simulink model "Sim_13_forh"  (R2019b)
settings: Solver=FixedStepAuto  StartTime=0.0  StopTime=sim_time  FixedStep=0.01  MaxStep=0.1  MinStep=0.0001  RelTol=0.01  AbsTol=0.01
values from neighbouring files (symbols this model uses):
  D = [ 0.66  0    0 ... (first row only)    [Sim_10_init.m]    (also in Sim_11_init.m; Sim_12_init.m; Sim_3_4_and_5_init.m; Sim_7_8_userdef_init.m)
  K_p = 0.08*[1.1  0    0 ... (first row only)    [Sim_10_init.m]    (also in Sim_11_init.m; Sim_12_init.m; Sim_3_4_and_5_init.m; Sim_7_8_userdef_init.m)
  K_v = 1*[10   0       0 ... (first row only)    [Sim_10_init.m]    (also in Sim_11_init.m; Sim_12_init.m; Sim_3_4_and_5_init.m; Sim_7_8_userdef_init.m = 3*[10   0       0)
  L1 = 10*diag([1 1 1])    [Sim_10_init.m]    (also in Sim_11_init.m; Sim_12_init.m; Sim_3_4_and_5_init.m; Sim_7_8_userdef_init.m)
  L2 = 20*M*diag([1 1 1])    [Sim_10_init.m]    (also in Sim_11_init.m; Sim_12_init.m; Sim_3_4_and_5_init.m = 10*M*diag([1 1 1]); Sim_7_8_userdef_init.m)
  L3 = 0.1*L2    [Sim_10_init.m]    (also in Sim_11_init.m; Sim_12_init.m; Sim_3_4_and_5_init.m; Sim_7_8_userdef_init.m)
  M = [ 16    0      0 ... (first row only)    [Sim_10_init.m]    (also in Sim_11_init.m; Sim_12_init.m; Sim_3_4_and_5_init.m; Sim_7_8_userdef_init.m)
  M_1 = inv(M)    [Sim_10_init.m]    (also in Sim_11_init.m; Sim_12_init.m; Sim_3_4_and_5_init.m; Sim_7_8_userdef_init.m)
  mu = 0.09    [Sim_10_init.m]    (also in Sim_11_init.m; Sim_12_init.m; Sim_3_4_and_5_init.m; Sim_7_8_userdef_init.m)
  path_planner_data = [start_pos; end_pos; Radius; Center]    [Sim_10_init.m]    (also in Sim_11_init.m; Sim_12_init.m; Sim_3_4_and_5_init.m; Sim_7_8_userdef_init.m)
  pathparameter = 0    [Sim_10_init.m]    (also in Sim_11_init.m = 1; Sim_12_init.m; Sim_3_4_and_5_init.m = 1; Sim_7_8_userdef_init.m = 1)
  start_pos = [10; 20; pi/2 ]    [Sim_10_init.m]    (also in Sim_11_init.m = [0; 0; 0 ]; Sim_12_init.m = [0; 0; 0 ]; Sim_3_4_and_5_init.m = [0; 0; 0 ]; Sim_7_init.m = [0; 0; 0 ])
undefined symbols (not defined in the file or in its folder): eta_set, p, start_time, t1, t2, t3, time
(part 1 of 3)
settings Model: Creator=einarsu  LastModifiedBy=yngve
settings SolverCC: InitialStep=0.01
settings DataIOCC: ReturnWorkspaceOutputs=off
settings OptimizationCC: LifeSpan=inf
settings DebuggingCC: SFExecutionAtInitializationDiag=none  ArithmeticOperatorsInVariantConditions=warning
settings SFSimCC: SimUseLocalCustomCode=off  CustomCodeUndefinedFunction=UseInterfaceOnly
settings RTWCC: RTWUseLocalCustomCode=off
settings CodeAppCC: StateflowObjectComments=on

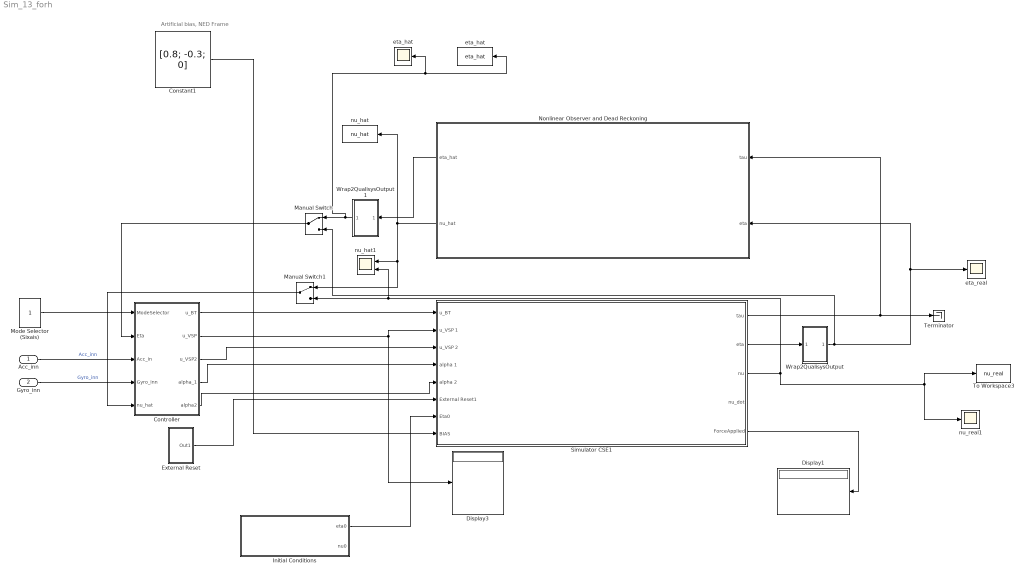
== system Sim_13_forh ==
  note: Artificial bias, NED Frame
  Acc_inn : Inport
  Gyro_inn : Inport  Port=2
  Constant1 : Constant  Value=[0.8; -0.3; 0]
  Controller : Subsystem
  Display1 : Display
  Display3 : Display
  External Reset : Subsystem
  "Initial Conditions " : Subsystem
  Manual Switch : ManualSwitch
  Manual Switch1 : ManualSwitch
  Mode Selector (Sixais) : Constant
  Nonlinear Observer and Dead Reckoning : Subsystem
  Simulator CSE1 : Subsystem
  Terminator : Terminator
  To Workspace3 : ToWorkspace  VariableName=nu_real  SaveFormat=Timeseries  SampleTime=-1
  "Wrap2QualisysOutput " : Subsystem
  Wrap2QualisysOutput 1 : Subsystem
  eta_hat : ToWorkspace  VariableName=eta_hat  SaveFormat=Timeseries  SampleTime=-1
  "eta_hat " : Scope
  "eta_real " : Scope
  nu_hat : ToWorkspace  VariableName=nu_hat  SaveFormat=Structure With Time  SampleTime=-1
  "nu_hat1 " : Scope  NumInputPorts=2
  "nu_real1 " : Scope
  wires:
  Controller/1(u_BT) -> Simulator CSE1/1(u_BT)
  Controller/4(alpha_1) -> Simulator CSE1/4(alpha 1)
  Controller/2(u_VSP) -> Simulator CSE1/2(u_VSP 1), Display3/1
  Controller/5(alpha2) -> Simulator CSE1/5(alpha 2)
  Controller/3("u_VSP2 ") -> Simulator CSE1/3(u_VSP 2)
  External Reset/1(Out1) -> Simulator CSE1/6(External Reset1)
  "Initial Conditions "/1(eta0) -> Simulator CSE1/7(Eta0)
  Mode Selector (Sixais)/1 -> Controller/1(ModeSelector)
  Simulator CSE1/2(eta) -> "Wrap2QualisysOutput "/1(In1)
  Acc_inn/1 -> Controller/3(Acc_in)  "Acc_inn"
  Gyro_inn/1 -> Controller/4(Gyro_inn)  "Gyro_inn"
  Simulator CSE1/5(ForceApplied) -> Display1/1
  Constant1/1 -> Simulator CSE1/8(BIAS)
  Nonlinear Observer and Dead Reckoning/1(eta_hat) -> Wrap2QualisysOutput 1/1(In1)
  Nonlinear Observer and Dead Reckoning/2(nu_hat) -> nu_hat/1, "nu_hat1 "/1, Manual Switch1/1
  Simulator CSE1/3(nu) -> To Workspace3/1, "nu_real1 "/1, Manual Switch1/2, "nu_hat1 "/2
  Simulator CSE1/1(tau) -> Terminator/1, Nonlinear Observer and Dead Reckoning/1(tau)
  "Wrap2QualisysOutput "/1(Out1) -> Manual Switch/2, "eta_real "/1, Nonlinear Observer and Dead Reckoning/2(eta)
  Manual Switch/1 -> Controller/2(Eta)
  Wrap2QualisysOutput 1/1(Out1) -> eta_hat/1, "eta_hat "/1, Manual Switch/1
  Manual Switch1/1 -> Controller/5("nu_hat ")

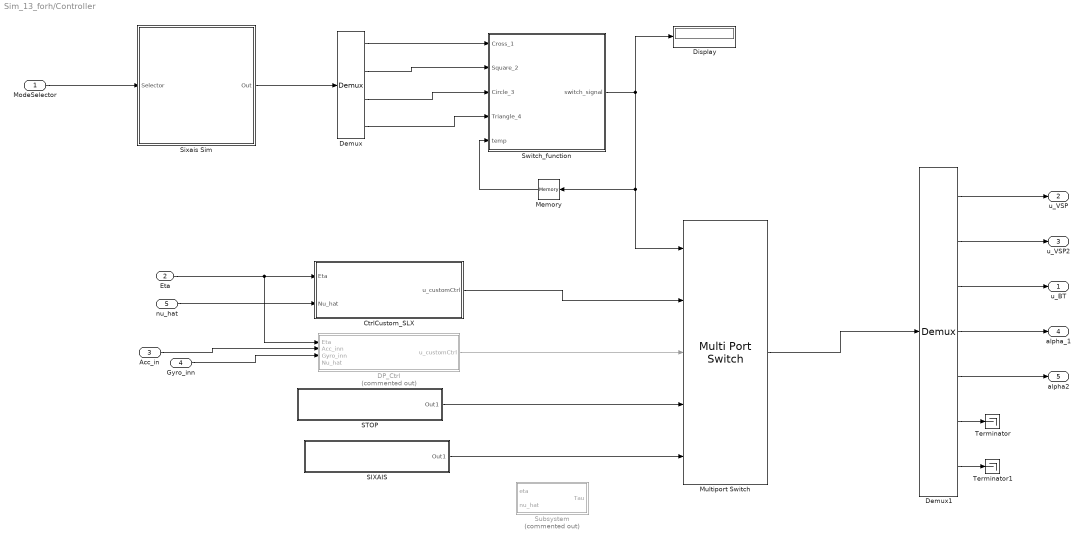
== system Sim_13_forh/Controller ==
  ModeSelector : Inport
  Eta : Inport  Port=2
  Acc_in : Inport  Port=3
  Gyro_inn : Inport  Port=4
  "nu_hat " : Inport  Port=5
  CtrlCustom_SLX : Subsystem
  DP_Ctrl : Subsystem  Commented=on
  Demux : Demux
  Demux1 : Demux  Outputs=7
  Display : Display
  Memory : Memory  InitialCondition=4
  Multiport Switch : MultiPortSwitch  Inputs=4
  SIXAIS : Subsystem
  STOP : Subsystem
  Sixais Sim : MATLAB Function  TreatAsAtomicUnit=on
  Subsystem : Subsystem  Commented=on
  Switch_function : MATLAB Function  TreatAsAtomicUnit=on
  Terminator : Terminator
  Terminator1 : Terminator
  u_BT : Outport  VectorParamsAs1DForOutWhenUnconnected=off
  u_VSP : Outport  Port=2  VectorParamsAs1DForOutWhenUnconnected=off
  "u_VSP2 " : Outport  Port=3  VectorParamsAs1DForOutWhenUnconnected=off
  alpha_1 : Outport  Port=4  VectorParamsAs1DForOutWhenUnconnected=off
  alpha2 : Outport  Port=5  VectorParamsAs1DForOutWhenUnconnected=off
  wires:
  Switch_function/1(switch_signal) -> Multiport Switch/1, Memory/1, Display/1
  Memory/1 -> Switch_function/5(temp)
  CtrlCustom_SLX/1(u_customCtrl) -> Multiport Switch/2
  Demux/1 -> Switch_function/1(Cross_1)
  Demux/2 -> Switch_function/2(Square_2)
  Demux/3 -> Switch_function/3(Circle_3)
  Demux/4 -> Switch_function/4(Triangle_4)
  Sixais Sim/1(Out) -> Demux/1
  ModeSelector/1 -> Sixais Sim/1(Selector)
  DP_Ctrl/1(u_customCtrl) -> Multiport Switch/3
  STOP/1(Out1) -> Multiport Switch/4
  SIXAIS/1(Out1) -> Multiport Switch/5
  Eta/1 -> DP_Ctrl/1(Eta), CtrlCustom_SLX/1(Eta)
  Acc_in/1 -> DP_Ctrl/2(Acc_inn)
  Gyro_inn/1 -> DP_Ctrl/3(Gyro_inn)
  Multiport Switch/1 -> Demux1/1
  Demux1/1 -> u_VSP/1
  Demux1/2 -> "u_VSP2 "/1
  Demux1/3 -> u_BT/1
  Demux1/4 -> alpha_1/1
  Demux1/5 -> alpha2/1
  Demux1/6 -> Terminator/1
  Demux1/7 -> Terminator1/1
  "nu_hat "/1 -> CtrlCustom_SLX/2(Nu_hat)

== system Sim_13_forh/External Reset ==
  note: Most relevant for Real-Time Simulations...
  Constant : Constant  Value=0
  Out1 : Outport  VectorParamsAs1DForOutWhenUnconnected=off
  wires:
  Constant/1 -> Out1/1

== system Sim_13_forh/Initial Conditions  ==
  Eta0 : Constant  Value=start_pos
  "V0 " : Constant  Value=zeros(3,1)
  eta0 : Outport  VectorParamsAs1DForOutWhenUnconnected=off
  nu0 : Outport  Port=2  VectorParamsAs1DForOutWhenUnconnected=off
  wires:
  "V0 "/1 -> nu0/1
  Eta0/1 -> eta0/1

== system Sim_13_forh/Nonlinear Observer and Dead Reckoning ==
  tau : Inport
  eta : Inport  Port=2
  Dead Reckoning : Subsystem
  Nonlinear Observer : Subsystem
  Scope : Scope
  eta_hat : Outport  VectorParamsAs1DForOutWhenUnconnected=off
  nu_hat : Outport  Port=2  VectorParamsAs1DForOutWhenUnconnected=off
  wires:
  Nonlinear Observer/1(eta_hat) -> Dead Reckoning/1(Eta_hat), eta_hat/1  "eta_hat"
  tau/1 -> Nonlinear Observer/2(tau)  "Tau"
  Nonlinear Observer/2(nu_hat) -> nu_hat/1
  Dead Reckoning/1(eta_out) -> Nonlinear Observer/1("eta_out_from_deadreck "), Scope/1
  eta/1 -> Dead Reckoning/2(eta)  "True Eta"

== system Sim_13_forh/Simulator CSE1 ==
  u_BT : Inport
  u_VSP 1 : Inport  Port=2
  u_VSP 2 : Inport  Port=3
  alpha 1 : Inport  Port=4
  alpha 2 : Inport  Port=5
  External Reset1 : Inport  Port=6
  Eta0 : Inport  Port=7
  BIAS : Inport  Port=8
  B Command to force mapping : Subsystem
  Display : Display
  Display1 : Display
  EquationsOfMotion (Fossen Model) : Subsystem
  Mux2 : Mux  Inputs=3
  tau : Outport  VectorParamsAs1DForOutWhenUnconnected=off
  eta : Outport  Port=2  VectorParamsAs1DForOutWhenUnconnected=off
  nu : Outport  Port=3  VectorParamsAs1DForOutWhenUnconnected=off
  nu_dot : Outport  Port=4  VectorParamsAs1DForOutWhenUnconnected=off
  ForceApplied : Outport  Port=5  VectorParamsAs1DForOutWhenUnconnected=off
  wires:
  alpha 2/1 -> B Command to force mapping/5(alpha 2)
  B Command to force mapping/2("F_y ") -> Mux2/2
  B Command to force mapping/1(F_x) -> Mux2/1
  u_VSP 1/1 -> B Command to force mapping/2(u_VSP 1), Display1/1
  alpha 1/1 -> B Command to force mapping/3(alpha 1)
  u_BT/1 -> B Command to force mapping/1(u_BT), Display/1
  u_VSP 2/1 -> B Command to force mapping/6(u_VSP 2)
  EquationsOfMotion (Fossen Model)/2(nuOut) -> B Command to force mapping/4(nu), EquationsOfMotion (Fossen Model)/4(nuInn), nu/1
  Eta0/1 -> EquationsOfMotion (Fossen Model)/1("[eta0] ")
  External Reset1/1 -> EquationsOfMotion (Fossen Model)/2(External Reset)
  EquationsOfMotion (Fossen Model)/1(EtaOut) -> eta/1
  EquationsOfMotion (Fossen Model)/3(nudot) -> nu_dot/1
  B Command to force mapping/3("MOMENT ") -> Mux2/3
  BIAS/1 -> EquationsOfMotion (Fossen Model)/5(Aritifiicial BIas)
  Mux2/1 -> ForceApplied/1, tau/1, EquationsOfMotion (Fossen Model)/3(tau)

== system Sim_13_forh/Wrap2QualisysOutput  ==
  In1 : Inport
  Demux : Demux  Outputs=3
  Gain : Gain  Gain=1000
  Gain1 : Gain  Gain=1000
  Gain2 : Gain  Gain=180/pi
  Mux : Mux  Inputs=3
  Wrap2psi : MATLAB Function  TreatAsAtomicUnit=on
  Out1 : Outport  VectorParamsAs1DForOutWhenUnconnected=off
  wires:
  Mux/1 -> Out1/1
  In1/1 -> Demux/1
  Demux/3 -> Wrap2psi/1(u)
  Demux/1 -> Gain/1
  Demux/2 -> Gain1/1
  Gain/1 -> Mux/1
  Gain1/1 -> Mux/2
  Gain2/1 -> Mux/3
  Wrap2psi/1(yQualisus) -> Gain2/1

== system Sim_13_forh/Wrap2QualisysOutput 1 ==
  In1 : Inport
  Demux : Demux  Outputs=3
  Gain : Gain  Gain=1000
  Gain1 : Gain  Gain=1000
  Gain2 : Gain  Gain=180/pi
  Mux : Mux  Inputs=3
  Wrap2psi : MATLAB Function  TreatAsAtomicUnit=on
  Out1 : Outport  VectorParamsAs1DForOutWhenUnconnected=off
  wires:
  Mux/1 -> Out1/1
  In1/1 -> Demux/1
  Demux/3 -> Wrap2psi/1(u)
  Demux/1 -> Gain/1
  Demux/2 -> Gain1/1
  Gain/1 -> Mux/1
  Gain1/1 -> Mux/2
  Gain2/1 -> Mux/3
  Wrap2psi/1(yQualisus) -> Gain2/1

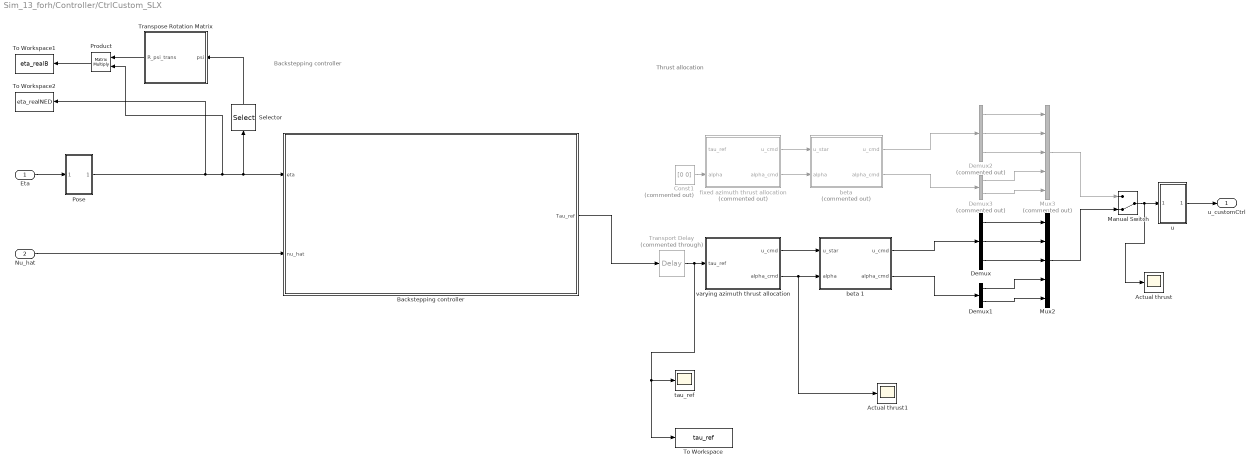
== system Sim_13_forh/Controller/CtrlCustom_SLX ==
  note: Backstepping controller
  note: Thrust allocation
  Eta : Inport
  Nu_hat : Inport  Port=2
  Actual thrust : Scope
  Actual thrust1 : Scope
  Backstepping controller : Subsystem
  Const1 : Constant  Commented=on  Value=[0 0]
  Demux : Demux  Outputs=3
  Demux1 : Demux  Outputs=2
  Demux2 : Demux  Commented=on  Outputs=3
  Demux3 : Demux  Commented=on  Outputs=2
  Manual Switch : ManualSwitch  CurrentSetting=0
  Mux2 : Mux  Inputs=5
  Mux3 : Mux  Commented=on  Inputs=5
  Pose : Subsystem
  Product : Product  Multiplication=Matrix(*)
  Selector : Selector  InputPortWidth=3  IndexOptions=Index vector (dialog)  Indices=[3]  OutputSizes=1
  To Workspace : ToWorkspace  VariableName=tau_ref  SaveFormat=Timeseries  SampleTime=-1
  To Workspace1 : ToWorkspace  VariableName=eta_realB  SaveFormat=Timeseries  SampleTime=-1
  To Workspace2 : ToWorkspace  VariableName=eta_realNED  SaveFormat=Timeseries  SampleTime=-1
  Transport Delay : TransportDelay  Commented=through  DelayTime=50  InitialOutput=[0.1 0.1 0.1]
  Transpose Rotation Matrix : MATLAB Function  TreatAsAtomicUnit=on
  "beta " : MATLAB Function  Commented=on  TreatAsAtomicUnit=on
  beta 1 : MATLAB Function  TreatAsAtomicUnit=on
  "fixed azimuth thrust allocation " : MATLAB Function  Commented=on  TreatAsAtomicUnit=on
  "tau_ref " : Scope
  u : Subsystem
  varying azimuth thrust allocation : MATLAB Function  TreatAsAtomicUnit=on
  u_customCtrl : Outport  VectorParamsAs1DForOutWhenUnconnected=off
  wires:
  u/1(Out1) -> u_customCtrl/1
  Const1/1 -> "fixed azimuth thrust allocation "/2(alpha)
  "fixed azimuth thrust allocation "/2(alpha_cmd) -> "beta "/2(alpha)
  varying azimuth thrust allocation/1(u_cmd) -> beta 1/1(u_star)
  "fixed azimuth thrust allocation "/1(u_cmd) -> "beta "/1(u_star)
  Manual Switch/1 -> Actual thrust/1, u/1(In1)
  beta 1/1(u_cmd) -> Demux/1
  Demux1/2 -> Mux2/5
  beta 1/2(alpha_cmd) -> Demux1/1
  Demux1/1 -> Mux2/4
  Demux/3 -> Mux2/3
  Demux/2 -> Mux2/2
  Demux/1 -> Mux2/1
  Demux3/2 -> Mux3/5
  Demux3/1 -> Mux3/4
  "beta "/2(alpha_cmd) -> Demux3/1
  Demux2/3 -> Mux3/3
  "beta "/1(u_cmd) -> Demux2/1
  Demux2/2 -> Mux3/2
  Demux2/1 -> Mux3/1
  Mux2/1 -> Manual Switch/2
  Mux3/1 -> Manual Switch/1
  Nu_hat/1 -> Backstepping controller/2(nu_hat)
  Pose/1(QTM) -> To Workspace2/1, Product/2, Selector/1, Backstepping controller/1(eta)
  Transpose Rotation Matrix/1(R_psi_trans) -> Product/1
  Product/1 -> To Workspace1/1
  Eta/1 -> Pose/1(eta)
  Selector/1 -> Transpose Rotation Matrix/1(psi)
  varying azimuth thrust allocation/2(alpha_cmd) -> Actual thrust1/1, beta 1/2(alpha)
  Backstepping controller/1("Tau_ref ") -> Transport Delay/1
  Transport Delay/1 -> To Workspace/1, "tau_ref "/1, varying azimuth thrust allocation/1(tau_ref)

== system Sim_13_forh/Controller/DP_Ctrl ==
  Eta : Inport
  Acc_inn : Inport  Port=2
  Gyro_inn : Inport  Port=3
  Nu_hat : Inport  Port=4
  Backstepping controller : Subsystem
  Constant : Constant  Value=[1;0;0]
  IMU (Consider if going to be properly Simulated...) : Subsystem
  Manual Switch : ManualSwitch  CurrentSetting=0
  Pose : Subsystem
  "Thrust Allocation " : Subsystem
  u : Subsystem
  u_customCtrl : Outport  VectorParamsAs1DForOutWhenUnconnected=off
  wires:
  Gyro_inn/1 -> IMU (Consider if going to be properly Simulated...)/1(Gyro_inn)
  Acc_inn/1 -> IMU (Consider if going to be properly Simulated...)/2(Acc_inn)
  Eta/1 -> Pose/1(eta)
  u/1(Out1) -> u_customCtrl/1
  IMU (Consider if going to be properly Simulated...)/2(Gyro) -> ?
  IMU (Consider if going to be properly Simulated...)/1(Acc) -> ?
  Constant/1 -> Manual Switch/1
  Manual Switch/1 -> "Thrust Allocation "/1(Tau_ref)
  "Thrust Allocation "/1(u_customCtrl) -> u/1(In1)
  Nu_hat/1 -> Backstepping controller/2(nu_hat)
  Pose/1(QTM) -> Backstepping controller/1(eta)
  Backstepping controller/1(Tau) -> Manual Switch/2

== system Sim_13_forh/Controller/SIXAIS ==
  Constant{,1..6} (7 alike) : Constant  Value=0
  Sixais Controller Not Simulated in Simulink : Subsystem
  Out1 : Outport  VectorParamsAs1DForOutWhenUnconnected=off
  wires:
  Constant/1 -> Sixais Controller Not Simulated in Simulink/1(In1)
  Constant1/1 -> Sixais Controller Not Simulated in Simulink/2(In2)
  Constant2/1 -> Sixais Controller Not Simulated in Simulink/3(In3)
  Constant3/1 -> Sixais Controller Not Simulated in Simulink/4(In4)
  Constant4/1 -> Sixais Controller Not Simulated in Simulink/5(In5)
  Constant5/1 -> Sixais Controller Not Simulated in Simulink/6(In6)
  Constant6/1 -> Sixais Controller Not Simulated in Simulink/7(In7)
  Sixais Controller Not Simulated in Simulink/1(Out1) -> Out1/1

== system Sim_13_forh/Controller/STOP ==
  Constant{,1..6} (7 alike) : Constant  Value=0
  Mux1 : Mux  Inputs=7
  Out1 : Outport  VectorParamsAs1DForOutWhenUnconnected=off
  wires:
  Mux1/1 -> Out1/1
  Constant/1 -> Mux1/1
  Constant1/1 -> Mux1/2
  Constant2/1 -> Mux1/3
  Constant3/1 -> Mux1/4
  Constant4/1 -> Mux1/5
  Constant5/1 -> Mux1/6
  Constant6/1 -> Mux1/7

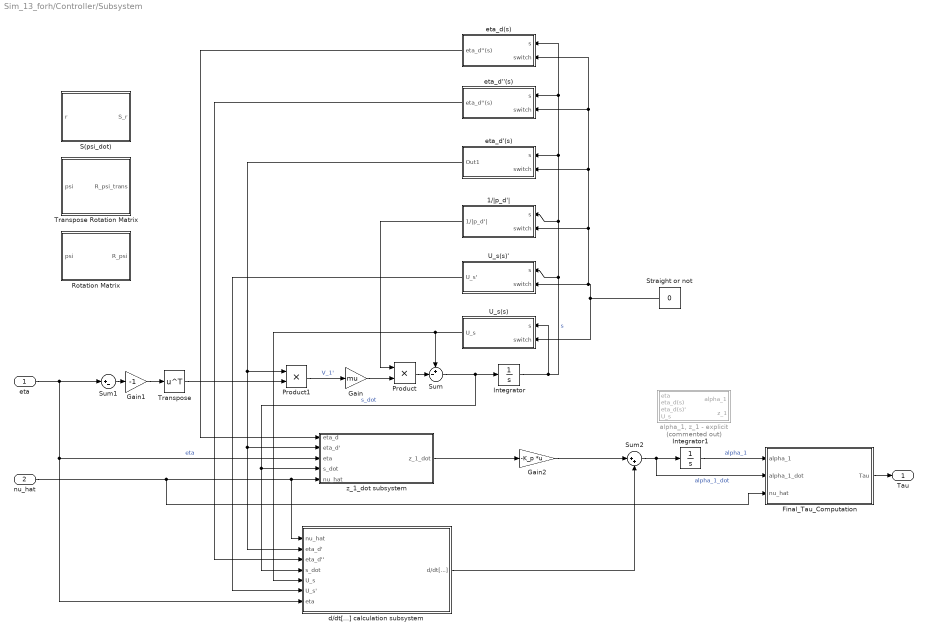
== system Sim_13_forh/Controller/Subsystem ==
  eta : Inport
  nu_hat : Inport  Port=2
  1/|p_d'| : Subsystem
  Final_Tau_Computation : Subsystem
  Gain : Gain  Gain=mu
  Gain1 : Gain  Gain=-1
  Gain2 : Gain  Gain=-K_p  Multiplication=Matrix(K*u)
  Integrator : Integrator
  Integrator1 : Integrator
  Product : Product
  Product1 : Product
  Rotation Matrix : MATLAB Function  TreatAsAtomicUnit=on
  S(psi_dot) : MATLAB Function  TreatAsAtomicUnit=on
  Straight or not : Constant  Value=0
  Sum : Sum  Inputs=+-|
  Sum1 : Sum  Inputs=|+-
  Sum2 : Sum  Inputs=|++
  Transpose : Math  Operator=transpose  SignedPower=off  SaturateOnIntegerOverflow=on
  Transpose Rotation Matrix : MATLAB Function  TreatAsAtomicUnit=on
  U_s(s) : Subsystem
  U_s(s)' : Subsystem
  "alpha_1, z_1 - explicit " : Subsystem  Commented=on
  d/dt[...] calculation subsystem : Subsystem
  eta_d''(s) : Subsystem
  eta_d'(s) : Subsystem
  eta_d(s) : Subsystem
  "z_1_dot subsystem " : Subsystem
  Tau : Outport
  wires:
  Integrator/1 -> U_s(s)'/1(s), 1/|p_d'|/1(s), eta_d'(s)/1(s), eta_d(s)/1(s), eta_d''(s)/1(s), U_s(s)/1(s)  "s"
  Sum/1 -> "z_1_dot subsystem "/4(s_dot), d/dt[...] calculation subsystem/4(s_dot), Integrator/1  "s_dot"
  U_s(s)/1(U_s) -> Sum/1, d/dt[...] calculation subsystem/5(U_s)
  Gain/1 -> Product/2
  Product/1 -> Sum/2
  1/|p_d'|/1(1/|p_d'|) -> Product/1
  eta_d'(s)/1(Out1) -> Product1/1, d/dt[...] calculation subsystem/2(eta_d'), "z_1_dot subsystem "/2(eta_d')
  Product1/1 -> Gain/1  "V_1'"
  Sum1/1 -> Gain1/1
  eta/1 -> "z_1_dot subsystem "/3(eta), d/dt[...] calculation subsystem/7("eta "), Sum1/1  "eta"
  ? -> Sum1/2  "eta_d"
  Gain1/1 -> Transpose/1
  Transpose/1 -> Product1/2
  "z_1_dot subsystem "/1(z_1_dot) -> Gain2/1
  Gain2/1 -> Sum2/1
  d/dt[...] calculation subsystem/1(d/dt[...]) -> Sum2/2
  Sum2/1 -> Final_Tau_Computation/2(alpha_1_dot), Integrator1/1  "alpha_1_dot"
  nu_hat/1 -> Final_Tau_Computation/3(nu_hat), d/dt[...] calculation subsystem/1(nu_hat), "z_1_dot subsystem "/5(nu_hat)
  Integrator1/1 -> Final_Tau_Computation/1(alpha_1)  "alpha_1"
  Final_Tau_Computation/1(Tau) -> Tau/1
  U_s(s)'/1(U_s') -> d/dt[...] calculation subsystem/6("U_s' ")
  Straight or not/1 -> U_s(s)/2(switch), eta_d(s)/2(switch), eta_d''(s)/2(switch), eta_d'(s)/2(switch), 1/|p_d'|/2(switch), U_s(s)'/2("switch ")
  eta_d''(s)/1("eta_d''(s) ") -> d/dt[...] calculation subsystem/3(eta_d'')
  eta_d(s)/1("eta_d''(s) ") -> "z_1_dot subsystem "/1(eta_d)

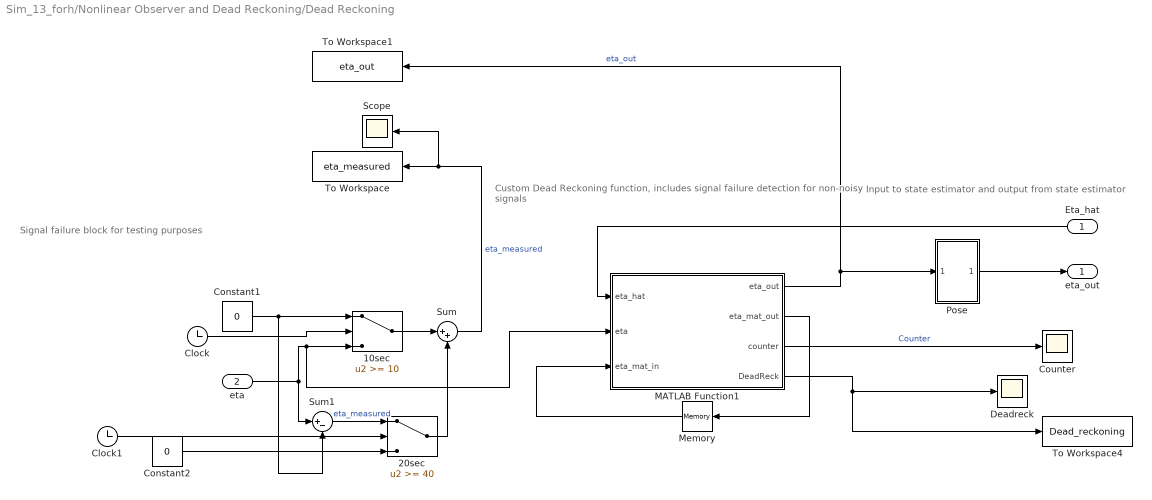
== system Sim_13_forh/Nonlinear Observer and Dead Reckoning/Dead Reckoning ==
  note: Custom Dead Reckoning function, includes signal failure
      | detection for non-noisy signals
  note: Input to state estimator and output from state estimator
  note: Signal failure block for testing purposes
  Eta_hat : Inport
  eta : Inport  Port=2
  10sec : Switch  Threshold=10
  "20sec " : Switch  Threshold=40
  Clock : Clock
  Clock1 : Clock
      settings: Decimation=20
  Constant1 : Constant  Value=0
  Constant2 : Constant  Value=0
  Counter : Scope
  "Deadreck " : Scope
  MATLAB Function1 : MATLAB Function  TreatAsAtomicUnit=on
  Memory : Memory  InitialCondition=zeros(4,3)  InheritSampleTime=on
  Pose : Subsystem
  Scope : Scope
  Sum : Sum  Inputs=|++
  Sum1 : Sum  Inputs=|+-
  To Workspace : ToWorkspace  VariableName=eta_measured  SaveFormat=Timeseries  SampleTime=-1
  To Workspace1 : ToWorkspace  VariableName=eta_out  SampleTime=-1
  To Workspace4 : ToWorkspace  VariableName=Dead_reckoning  SaveFormat=Timeseries  SampleTime=-1
  eta_out : Outport
  wires:
  MATLAB Function1/2(eta_mat_out) -> Memory/1
  Sum/1 -> Scope/1, To Workspace/1  "eta_measured"
  Eta_hat/1 -> MATLAB Function1/1(eta_hat)
  MATLAB Function1/1(eta_out) -> Pose/1(eta), To Workspace1/1  "eta_out"
  Clock1/1 -> "20sec "/2
  Constant1/1 -> Sum1/2, 10sec/1
  Constant2/1 -> "20sec "/3
  MATLAB Function1/4(DeadReck) -> To Workspace4/1, "Deadreck "/1
  "20sec "/1 -> Sum/2
  10sec/1 -> Sum/1
  Memory/1 -> MATLAB Function1/3(eta_mat_in)
  Clock/1 -> 10sec/2
  MATLAB Function1/3(counter) -> Counter/1  "Counter"
  eta/1 -> Sum1/1, MATLAB Function1/2(eta), 10sec/3
  Sum1/1 -> "20sec "/1  "eta_measured"
  Pose/1(QTM) -> eta_out/1

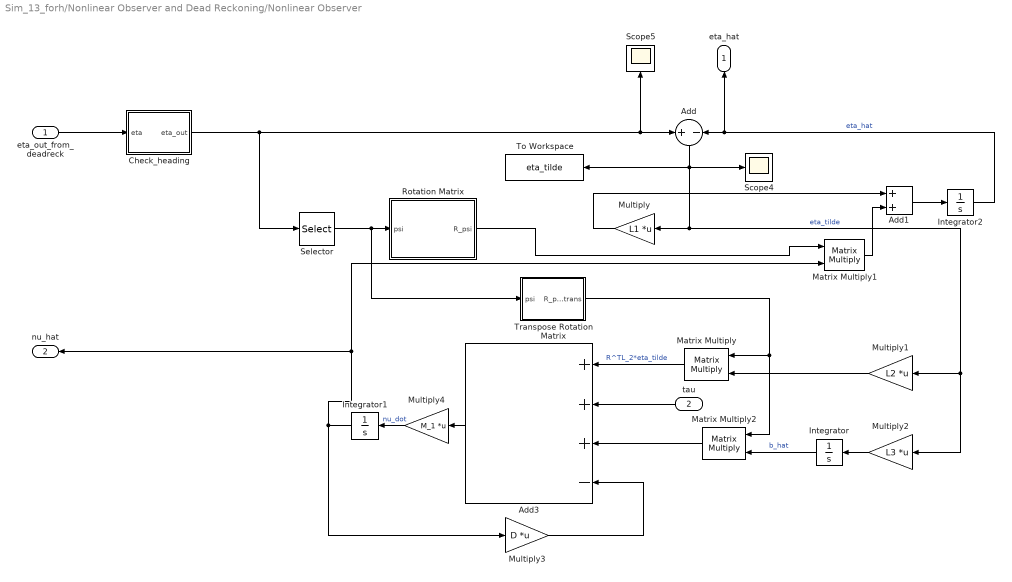
== system Sim_13_forh/Nonlinear Observer and Dead Reckoning/Nonlinear Observer ==
  "eta_out_from_deadreck " : Inport
  tau : Inport  Port=2
  Add : Sum  Inputs=+-
  Add1 : Sum
  Add3 : Sum  Inputs=+++-
  Check_heading : MATLAB Function  TreatAsAtomicUnit=on
  Integrator : Integrator
  Integrator1 : Integrator
  Integrator2 : Integrator
  Matrix Multiply : Product  Multiplication=Matrix(*)
  Matrix Multiply1 : Product  Multiplication=Matrix(*)
  Matrix Multiply2 : Product  Multiplication=Matrix(*)
  Multiply : Gain  Gain=L1  Multiplication=Matrix(K*u)
  Multiply1 : Gain  Gain=L2  Multiplication=Matrix(K*u)
  Multiply2 : Gain  Gain=L3  Multiplication=Matrix(K*u)
  Multiply3 : Gain  Gain=D  Multiplication=Matrix(K*u)
  Multiply4 : Gain  Gain=M_1  Multiplication=Matrix(K*u)
  Rotation Matrix : MATLAB Function  TreatAsAtomicUnit=on
  Scope4 : Scope
  Scope5 : Scope
  Selector : Selector  InputPortWidth=3  IndexOptions=Index vector (dialog)  Indices=3  OutputSizes=1
  To Workspace : ToWorkspace  VariableName=eta_tilde  SaveFormat=Timeseries  SampleTime=-1
  Transpose Rotation Matrix : MATLAB Function  TreatAsAtomicUnit=on
  eta_hat : Outport
  nu_hat : Outport  Port=2  VectorParamsAs1DForOutWhenUnconnected=off
  wires:
  Multiply/1 -> Add1/1
  Multiply2/1 -> Integrator/1
  Rotation Matrix/1(R_psi) -> Matrix Multiply1/1
  Multiply1/1 -> Matrix Multiply/2
  Matrix Multiply/1 -> Add3/1  "R^TL_2*eta_tilde"
  "eta_out_from_deadreck "/1 -> Check_heading/1(eta)
  Matrix Multiply1/1 -> Add1/2
  Add/1 -> Scope4/1, Multiply/1, Multiply1/1, Multiply2/1, To Workspace/1  "eta_tilde"
  Multiply4/1 -> Integrator1/1  "nu_dot"
  Selector/1 -> Transpose Rotation Matrix/1(psi), Rotation Matrix/1(psi)
  Integrator2/1 -> Add/2, eta_hat/1  "eta_hat"
  Integrator/1 -> Matrix Multiply2/2  "b_hat"
  tau/1 -> Add3/2
  Matrix Multiply2/1 -> Add3/3
  Multiply3/1 -> Add3/4
  Add3/1 -> Multiply4/1
  Add1/1 -> Integrator2/1
  Integrator1/1 -> nu_hat/1, Matrix Multiply1/2, Multiply3/1
  Transpose Rotation Matrix/1(R_psi_trans) -> Matrix Multiply2/1, Matrix Multiply/1
  Check_heading/1(eta_out) -> Selector/1, Scope5/1, Add/1

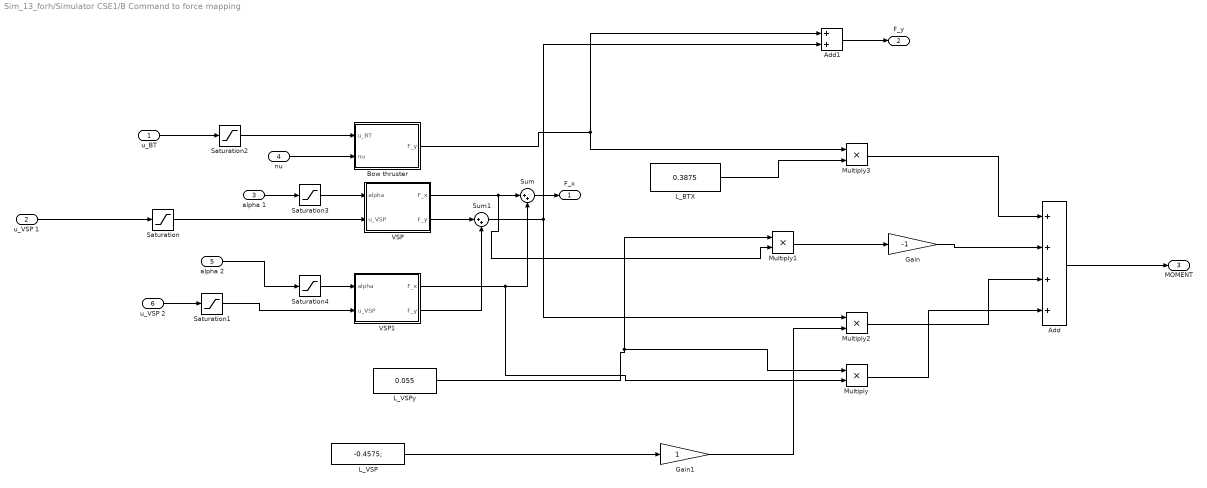
== system Sim_13_forh/Simulator CSE1/B Command to force mapping ==
  u_BT : Inport
  u_VSP 1 : Inport  Port=2
  alpha 1 : Inport  Port=3
  nu : Inport  Port=4
  alpha 2 : Inport  Port=5
  u_VSP 2 : Inport  Port=6
  Add : Sum  Inputs=++++
  Add1 : Sum
  Bow thruster : MATLAB Function  TreatAsAtomicUnit=on
  Gain : Gain  Gain=-1
  Gain1 : Gain
  L_BTX : Constant  Value=0.3875
  L_VSP : Constant  Value=-0.4575;
  L_VSPy : Constant  Value=0.055
  Multiply{,1..3} (4 alike) : Product
  Saturation : Saturate  UpperLimit=1  LowerLimit=0
  Saturation1 : Saturate  UpperLimit=1  LowerLimit=0
  Saturation2 : Saturate  UpperLimit=1  LowerLimit=-1
  Saturation3 : Saturate  UpperLimit=pi  LowerLimit=-pi
  Saturation4 : Saturate  UpperLimit=pi  LowerLimit=-pi
  Sum : Sum  Inputs=|++
  Sum1 : Sum  Inputs=|++
  VSP : MATLAB Function  TreatAsAtomicUnit=on
  VSP1 : MATLAB Function  TreatAsAtomicUnit=on
  F_x : Outport  VectorParamsAs1DForOutWhenUnconnected=off
  "F_y " : Outport  Port=2  VectorParamsAs1DForOutWhenUnconnected=off
  "MOMENT " : Outport  Port=3  VectorParamsAs1DForOutWhenUnconnected=off
  wires:
  alpha 1/1 -> Saturation3/1
  nu/1 -> Bow thruster/2(nu)
  Bow thruster/1(F_y) -> Add1/1, Multiply3/1
  VSP/2(F_y) -> Sum1/1
  Sum1/1 -> Add1/2, Multiply2/1
  VSP1/2(F_y) -> Sum1/2
  VSP1/1(F_x) -> Multiply/2, Sum/2
  VSP/1(F_x) -> Multiply1/2, Sum/1
  Sum/1 -> F_x/1
  alpha 2/1 -> Saturation4/1
  u_VSP 2/1 -> Saturation1/1
  L_VSP/1 -> Gain1/1
  L_BTX/1 -> Multiply3/2
  L_VSPy/1 -> Multiply/1, Multiply1/1
  Multiply3/1 -> Add/1
  Multiply1/1 -> Gain/1
  Multiply2/1 -> Add/3
  Multiply/1 -> Add/4
  Add/1 -> "MOMENT "/1
  Gain/1 -> Add/2
  Gain1/1 -> Multiply2/2
  Add1/1 -> "F_y "/1
  Saturation/1 -> VSP/2(u_VSP)
  Saturation1/1 -> VSP1/2(u_VSP)
  u_BT/1 -> Saturation2/1
  u_VSP 1/1 -> Saturation/1
  Saturation2/1 -> Bow thruster/1(u_BT)
  Saturation3/1 -> VSP/1(alpha)
  Saturation4/1 -> VSP1/1(alpha)

== system Sim_13_forh/Simulator CSE1/EquationsOfMotion (Fossen Model) ==
  "[eta0] " : Inport
  External Reset : Inport  Port=2
  tau : Inport  Port=3
  nuInn : Inport  Port=4
  Aritifiicial BIas : Inport  Port=5
  Add : Sum
  MATLAB Function : MATLAB Function  TreatAsAtomicUnit=on
  Position : Integrator  ExternalReset=either  InitialConditionSource=external  InitialCondition=[0 0 0]'
  Selector : Selector  InputPortWidth=3  IndexOptions=Index vector (dialog)  Indices=[3]  OutputSizes=1
  Velocity : Integrator  ExternalReset=either  InitialCondition=[0 0 0]'
  kinematics : MATLAB Function  TreatAsAtomicUnit=on
  kinetics : MATLAB Function  TreatAsAtomicUnit=on
  EtaOut : Outport  VectorParamsAs1DForOutWhenUnconnected=off
  nuOut : Outport  Port=2  VectorParamsAs1DForOutWhenUnconnected=off
  nudot : Outport  Port=3  VectorParamsAs1DForOutWhenUnconnected=off
  wires:
  tau/1 -> Add/1
  Position/1 -> EtaOut/1, Selector/1, kinematics/2(eta)
  "[eta0] "/1 -> Position/3
  nuInn/1 -> kinetics/2(nu)
  kinematics/1(eta_dot) -> Position/1
  Velocity/1 -> nuOut/1, kinematics/1(nu)
  kinetics/1(nu_dot) -> nudot/1, Velocity/1
  External Reset/1 -> Velocity/2, Position/2
  Add/1 -> kinetics/1(tau)
  Aritifiicial BIas/1 -> MATLAB Function/2(NedVector)
  Selector/1 -> MATLAB Function/1(psi)
  MATLAB Function/1(BodyVector) -> Add/2

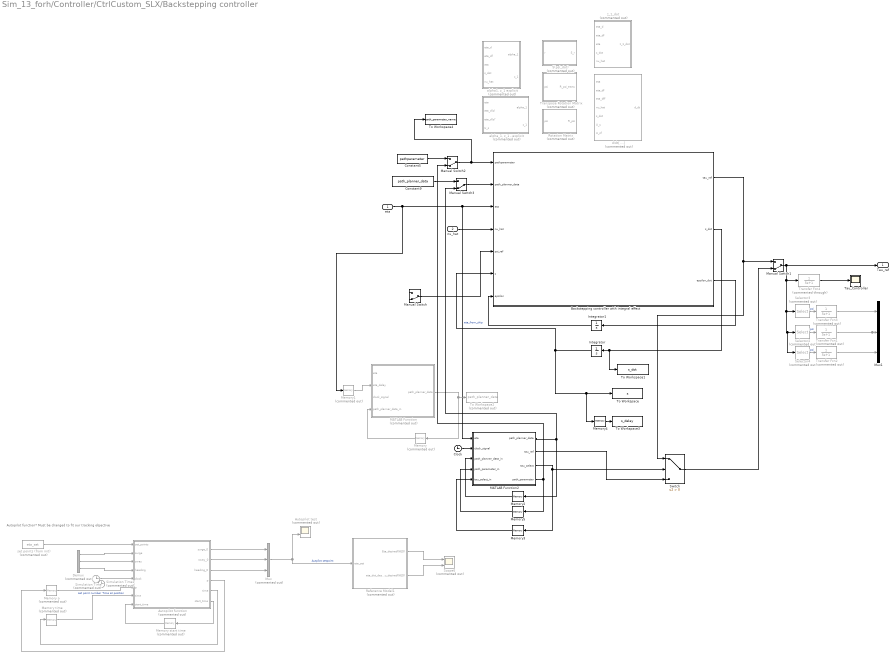
== system Sim_13_forh/Controller/CtrlCustom_SLX/Backstepping controller ==
  note: Autopilot function* Must be changed to fit our tracking objective
  eta : Inport
  nu_hat : Inport  Port=2
  "Autopilot function " : MATLAB Function  Commented=on  TreatAsAtomicUnit=on
  "Autopilot test " : Scope  Commented=on  NumInputPorts=2
  "Backstepping controller with integral effect " : MATLAB Function  TreatAsAtomicUnit=on  SystemSampleTime=0.1
  Clock : Clock
  Constant5 : Constant  Value=pathparameter
  Constant9 : Constant  Value=path_planner_data
  Demux : Demux  Commented=on  Outputs=3
  Integrator : Integrator
  Integrator1 : Integrator  InitialCondition=[0;0;0]  LimitOutput=on  UpperSaturationLimit=1  LowerSaturationLimit=-1
  MATLAB Function : MATLAB Function  Commented=on  TreatAsAtomicUnit=on
  MATLAB Function2 : MATLAB Function  TreatAsAtomicUnit=on
  Manual Switch{,1..3} (4 alike) : ManualSwitch  CurrentSetting=0
  Memory : Memory  Commented=on
  Memory start time : Memory  Commented=on  InitialCondition=start_time  InheritSampleTime=on
  Memory p : Memory  Commented=on  InitialCondition=p  InheritSampleTime=on
  Memory time : Memory  Commented=on  InitialCondition=time
  Memory1 : Memory  Commented=on
  Memory{2..5} (4 alike) : Memory
  Mux : Mux  Commented=on  Inputs=3
  Mux1 : Mux  Inputs=3
  Reference Model1 : Subsystem  Commented=on
  Rotation Matrix : MATLAB Function  Commented=on  TreatAsAtomicUnit=on
  S(psi_dot) : MATLAB Function  Commented=on  TreatAsAtomicUnit=on
  Scope6 : Scope  Commented=on  NumInputPorts=2
  Selector2 : Selector  Commented=on  InputPortWidth=3  IndexOptions=Index vector (dialog)  Indices=[2]  OutputSizes=1
  Selector3 : Selector  Commented=on  InputPortWidth=3  IndexOptions=Index vector (dialog)  Indices=[1]  OutputSizes=1
  Selector4 : Selector  Commented=on  InputPortWidth=3  IndexOptions=Index vector (dialog)  Indices=[3]  OutputSizes=1
  Simulation Time : Clock  Commented=on
  Simulation Time1 : Clock  Commented=on
  Switch : Switch  Criteria=u2 > Threshold
  Tau_Controller : Scope
  To Workspace : ToWorkspace  VariableName=s  SaveFormat=Timeseries  SampleTime=-1
  To Workspace1 : ToWorkspace  VariableName=s_dot  SaveFormat=Timeseries  SampleTime=-1
  To Workspace2 : ToWorkspace  Commented=on  VariableName=path_planner_data  SaveFormat=Timeseries  SampleTime=-1
  To Workspace3 : ToWorkspace  VariableName=s_delay  SaveFormat=Timeseries  SampleTime=-1
  To Workspace4 : ToWorkspace  VariableName=path_parameter_name  SaveFormat=Timeseries  SampleTime=-1
  Transfer Fcn1 : TransferFcn  Commented=on  Denominator=[5 1]
  Transfer Fcn2 : TransferFcn  Commented=on  Denominator=[5 1]
  Transfer Fcn3 : TransferFcn  Commented=on  Denominator=[5 1]
  Transfer Fcn4 : TransferFcn  Commented=through  Denominator=[5 1]
  Transpose Rotation Matrix : MATLAB Function  Commented=on  TreatAsAtomicUnit=on
  "alpha1, z_1 explicit" : MATLAB Function  Commented=on  TreatAsAtomicUnit=on
  "alpha_1, z_1 - explicit " : Subsystem  Commented=on
  d/dt[....] : MATLAB Function  Commented=on  TreatAsAtomicUnit=on
  set points (from init) : Constant  Commented=on  Value=eta_set
  z_1_dot : MATLAB Function  Commented=on  TreatAsAtomicUnit=on
  "Tau_ref " : Outport
  wires:
  Constant9/1 -> Manual Switch3/1
  "Autopilot function "/6(start_time) -> Memory start time/1
  Memory time/1 -> "Autopilot function "/7("time ")  "Time at position"
  Memory start time/1 -> "Autopilot function "/8("start_time ")
  "Autopilot function "/3(heading_0) -> Mux/3
  "Autopilot function "/5(time) -> Memory time/1
  "Autopilot function "/1(surge_0) -> Mux/1
  Simulation Time/1 -> "Autopilot function "/5(clock)
  Demux/2 -> "Autopilot function "/3(sway)
  Demux/1 -> "Autopilot function "/2(surge)
  eta/1 -> Memory1/1, MATLAB Function2/1(eta), "Backstepping controller with integral effect "/3(eta)  "eta_from_ship"
  Demux/3 -> "Autopilot function "/4(heading)
  set points (from init)/1 -> "Autopilot function "/1(set_points)
  "Autopilot function "/2(sway_0) -> Mux/2
  "Autopilot function "/4(p) -> Memory p/1
  Mux/1 -> "Autopilot test "/2, Reference Model1/1("eta_set ")  "Autpilot setpoint"
  Memory p/1 -> "Autopilot function "/6("p ")  "set point number"
  Reference Model1/1(Eta_desired(NED)) -> Scope6/1
  Reference Model1/2(eta_dot_desired = nu_desired(NED)) -> Scope6/2
  Manual Switch1/1 -> Selector3/1, Selector2/1, Selector4/1, Transfer Fcn4/1, "Tau_ref "/1
  Manual Switch3/1 -> "Backstepping controller with integral effect "/2(path_planner_data)
  "Backstepping controller with integral effect "/3(epsilon_dot) -> Integrator1/1
  "Backstepping controller with integral effect "/2(s_dot) -> To Workspace1/1, Integrator/1
  Manual Switch/1 -> "Backstepping controller with integral effect "/5(psi_ref)
  nu_hat/1 -> "Backstepping controller with integral effect "/4(nu_hat)
  Integrator/1 -> Memory4/1, To Workspace/1, "Backstepping controller with integral effect "/6(s)
  Integrator1/1 -> "Backstepping controller with integral effect "/7(epsilon)
  Transfer Fcn1/1 -> Mux1/2
  Selector2/1 -> Transfer Fcn1/1  "psi"
  Selector4/1 -> Transfer Fcn2/1  "psi"
  Selector3/1 -> Transfer Fcn3/1  "psi"
  Transfer Fcn3/1 -> Mux1/1
  Transfer Fcn2/1 -> Mux1/3
  Transfer Fcn4/1 -> Tau_Controller/1
  MATLAB Function/1(path_planner_data) -> To Workspace2/1, Memory/1
  Memory/1 -> MATLAB Function/4(path_planner_data_in)
  Memory1/1 -> MATLAB Function/2(eta_delay)
  Clock/1 -> MATLAB Function2/2(clock_signal)
  MATLAB Function2/1(path_planner_data) -> Manual Switch3/2, Memory2/1
  Memory2/1 -> MATLAB Function2/3(path_planner_data_in)
  MATLAB Function2/3(tau_select) -> Memory3/1, Switch/2
  Memory3/1 -> MATLAB Function2/5(tau_select_in)
  MATLAB Function2/2(tau_ref) -> Switch/3
  "Backstepping controller with integral effect "/1(tau_ref) -> Manual Switch1/1, Switch/1
  Switch/1 -> Manual Switch1/2
  Memory4/1 -> To Workspace3/1
  MATLAB Function2/4(path_parameter) -> Memory5/1, Manual Switch2/2
  Constant5/1 -> Manual Switch2/1
  Manual Switch2/1 -> To Workspace4/1, "Backstepping controller with integral effect "/1(pathparameter)
  Memory5/1 -> MATLAB Function2/4(path_parameter_in)

== system Sim_13_forh/Controller/CtrlCustom_SLX/Pose ==
  eta : Inport
  Demux : Demux  Outputs=3
  Gain : Gain  Gain=1/1000
  Gain1 : Gain  Gain=1/1000
  Gain2 : Gain  Gain=180/pi
  Gain3 : Gain  Gain=pi/180
  MATLAB Function : MATLAB Function  Commented=on  TreatAsAtomicUnit=on
  Manual Switch : ManualSwitch
  Memory : Memory  Commented=on
  Mux : Mux  Inputs=3
  Wrap2psi : MATLAB Function  TreatAsAtomicUnit=on
  QTM : Outport  VectorParamsAs1DForOutWhenUnconnected=off
  wires:
  Demux/2 -> Gain1/1  "y_m"
  Demux/3 -> Gain3/1  "psi_m"
  Demux/1 -> Gain/1  "x_m"
  Mux/1 -> QTM/1
  eta/1 -> Demux/1
  ? -> Wrap2psi/1(u)
  Wrap2psi/1(yQualisus) -> Gain2/1
  Gain/1 -> Mux/1
  Gain1/1 -> Mux/2
  MATLAB Function/1(psi_out) -> Memory/1, Manual Switch/2
  Memory/1 -> MATLAB Function/2(psi_old)
  Gain3/1 -> MATLAB Function/1(psi), Manual Switch/1
  Manual Switch/1 -> Mux/3

== system Sim_13_forh/Controller/CtrlCustom_SLX/u ==
  In1 : Inport
  Constant : Constant  Value=0.3
  Constant1 : Constant  Value=0.3
  Demux1 : Demux  Outputs=5
  Mux : Mux  Inputs=7
  Saturation1 : Saturate  UpperLimit=1  LowerLimit=0
  Saturation11 : Saturate  UpperLimit=1  LowerLimit=0
  Out1 : Outport  VectorParamsAs1DForOutWhenUnconnected=off
  wires:
  In1/1 -> Demux1/1
  Demux1/1 -> Saturation11/1  "u_vsp1"
  Demux1/2 -> Saturation1/1  "u_VSP2"
  Demux1/3 -> Mux/3  "U_BT"
  Demux1/4 -> Mux/4  "alpha_VSP1"
  Demux1/5 -> Mux/5  "alpha_VSP2"
  Constant/1 -> Mux/6  "omega_VSP1"
  Constant1/1 -> Mux/7  "omega_VSP2"
  Mux/1 -> Out1/1
  Saturation11/1 -> Mux/1
  Saturation1/1 -> Mux/2

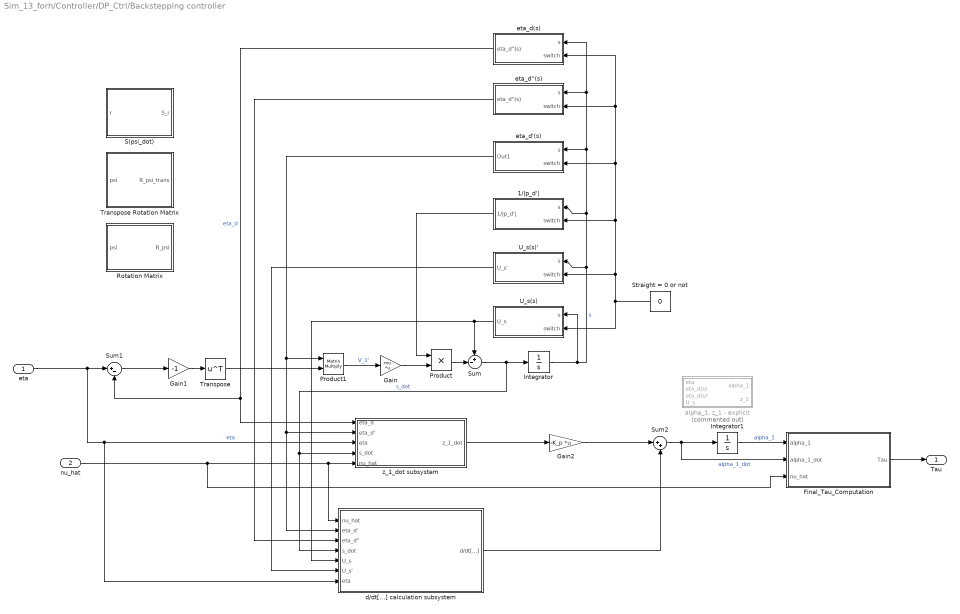
== system Sim_13_forh/Controller/DP_Ctrl/Backstepping controller ==
  eta : Inport
  nu_hat : Inport  Port=2
  1/|p_d'| : Subsystem
  Final_Tau_Computation : Subsystem
  Gain : Gain  Gain=mu  Multiplication=Matrix(K*u)
  Gain1 : Gain  Gain=-1
  Gain2 : Gain  Gain=-K_p  Multiplication=Matrix(K*u)
  Integrator : Integrator
  Integrator1 : Integrator
  Product : Product
  Product1 : Product  Multiplication=Matrix(*)
  Rotation Matrix : MATLAB Function  TreatAsAtomicUnit=on
  S(psi_dot) : MATLAB Function  TreatAsAtomicUnit=on
  Straight = 0 or not : Constant  Value=0
  Sum : Sum  Inputs=+-|
  Sum1 : Sum  Inputs=|+-
  Sum2 : Sum  Inputs=|++
  Transpose : Math  Operator=transpose  SignedPower=off  SaturateOnIntegerOverflow=on
  Transpose Rotation Matrix : MATLAB Function  TreatAsAtomicUnit=on
  U_s(s) : Subsystem
  U_s(s)' : Subsystem
  "alpha_1, z_1 - explicit " : Subsystem  Commented=on
  d/dt[...] calculation subsystem : Subsystem
  eta_d''(s) : Subsystem
  eta_d'(s) : Subsystem
  eta_d(s) : Subsystem
  "z_1_dot subsystem " : Subsystem
  Tau : Outport
  wires:
  Integrator/1 -> U_s(s)'/1(s), 1/|p_d'|/1(s), eta_d'(s)/1(s), eta_d(s)/1(s), eta_d''(s)/1(s), U_s(s)/1(s)  "s"
  Sum/1 -> "z_1_dot subsystem "/4(s_dot), d/dt[...] calculation subsystem/4(s_dot), Integrator/1  "s_dot"
  U_s(s)/1(U_s) -> d/dt[...] calculation subsystem/5(U_s), Sum/1
  Gain/1 -> Product/2
  Product/1 -> Sum/2
  1/|p_d'|/1(1/|p_d'|) -> Product/1
  Product1/1 -> Gain/1  "V_1'"
  Sum1/1 -> Gain1/1
  eta/1 -> Sum1/1, "z_1_dot subsystem "/3(eta), d/dt[...] calculation subsystem/7("eta ")  "eta"
  eta_d(s)/1("eta_d''(s) ") -> Sum1/2, "z_1_dot subsystem "/1(eta_d)  "eta_d"
  Gain1/1 -> Transpose/1
  Transpose/1 -> Product1/2
  "z_1_dot subsystem "/1(z_1_dot) -> Gain2/1
  Gain2/1 -> Sum2/1
  d/dt[...] calculation subsystem/1(d/dt[...]) -> Sum2/2
  Sum2/1 -> Final_Tau_Computation/2(alpha_1_dot), Integrator1/1  "alpha_1_dot"
  nu_hat/1 -> Final_Tau_Computation/3(nu_hat), d/dt[...] calculation subsystem/1(nu_hat), "z_1_dot subsystem "/5(nu_hat)
  Integrator1/1 -> Final_Tau_Computation/1(alpha_1)  "alpha_1"
  Final_Tau_Computation/1(Tau) -> Tau/1
  U_s(s)'/1(U_s') -> d/dt[...] calculation subsystem/6("U_s' ")
  Straight = 0 or not/1 -> U_s(s)/2(switch), eta_d(s)/2(switch), eta_d''(s)/2(switch), eta_d'(s)/2(switch), 1/|p_d'|/2(switch), U_s(s)'/2("switch ")
  eta_d''(s)/1("eta_d''(s) ") -> d/dt[...] calculation subsystem/3(eta_d'')
  eta_d'(s)/1(Out1) -> Product1/1, d/dt[...] calculation subsystem/2(eta_d'), "z_1_dot subsystem "/2(eta_d')

== system Sim_13_forh/Controller/DP_Ctrl/IMU (Consider if going to be properly Simulated...) ==
  Gyro_inn : Inport
  Acc_inn : Inport  Port=2
  Demux : Demux  Outputs=3
  Demux1 : Demux  Outputs=3
  Mux : Mux  Inputs=3
  Mux2 : Mux  Inputs=3
  Acc : Outport  VectorParamsAs1DForOutWhenUnconnected=off
  Gyro : Outport  Port=2  VectorParamsAs1DForOutWhenUnconnected=off
  wires:
  Acc_inn/1 -> Demux1/1
  Gyro_inn/1 -> Demux/1
  Demux/1 -> Mux2/1
  Demux/2 -> Mux2/2
  Demux/3 -> Mux2/3
  Demux1/2 -> Mux/2
  Demux1/3 -> Mux/3
  Mux2/1 -> Gyro/1
  Demux1/1 -> Mux/1
  Mux/1 -> Acc/1

== system Sim_13_forh/Controller/DP_Ctrl/Pose ==
  eta : Inport
  Demux : Demux  Outputs=3
  Mux : Mux  Inputs=3
  QTM : Outport  VectorParamsAs1DForOutWhenUnconnected=off
  wires:
  eta/1 -> Demux/1
  Mux/1 -> QTM/1
  Demux/1 -> Mux/1  "x_m"
  Demux/3 -> Mux/3  "psi_m"
  Demux/2 -> Mux/2  "y_m"

== system Sim_13_forh/Controller/DP_Ctrl/Thrust Allocation  ==
  Tau_ref : Inport
  Const1 : Constant  Value=[0 0]
  Demux : Demux  Outputs=3
  Demux1 : Demux  Outputs=2
  Demux2 : Demux  Outputs=3
  Demux3 : Demux  Outputs=2
  Manual Switch : ManualSwitch  CurrentSetting=0
  Mux2 : Mux  Inputs=5
  Mux3 : Mux  Inputs=5
  "beta " : MATLAB Function  TreatAsAtomicUnit=on
  beta 1 : MATLAB Function  TreatAsAtomicUnit=on
  "fixed azimuth thrust allocation " : MATLAB Function  TreatAsAtomicUnit=on
  u : Subsystem
  varying azimuth thrust allocation : MATLAB Function  TreatAsAtomicUnit=on
  u_customCtrl : Outport  VectorParamsAs1DForOutWhenUnconnected=off
  wires:
  beta 1/1(u_cmd) -> Demux/1
  Demux/1 -> Mux2/1
  Demux1/1 -> Mux2/4
  "fixed azimuth thrust allocation "/2(alpha_cmd) -> "beta "/2(alpha)
  Demux/2 -> Mux2/2
  Demux1/2 -> Mux2/5
  "beta "/1(u_cmd) -> Demux2/1
  Mux2/1 -> Manual Switch/2
  "beta "/2(alpha_cmd) -> Demux3/1
  beta 1/2(alpha_cmd) -> Demux1/1
  u/1(Out1) -> u_customCtrl/1
  Demux2/1 -> Mux3/1
  Manual Switch/1 -> u/1(In1)
  Demux2/2 -> Mux3/2
  Demux3/2 -> Mux3/5
  Tau_ref/1 -> "fixed azimuth thrust allocation "/1(tau_ref), varying azimuth thrust allocation/1(tau_ref)
  varying azimuth thrust allocation/1(u_cmd) -> beta 1/1(u_star)
  Demux/3 -> Mux2/3
  Demux2/3 -> Mux3/3
  varying azimuth thrust allocation/2(alpha_cmd) -> beta 1/2(alpha)
  Const1/1 -> "fixed azimuth thrust allocation "/2(alpha)
  Demux3/1 -> Mux3/4
  "fixed azimuth thrust allocation "/1(u_cmd) -> "beta "/1(u_star)
  Mux3/1 -> Manual Switch/1

== system Sim_13_forh/Controller/DP_Ctrl/u ==
  In1 : Inport
  Demux1 : Demux  Outputs=7
  Mux : Mux  Inputs=7
  Out1 : Outport  VectorParamsAs1DForOutWhenUnconnected=off
  wires:
  Mux/1 -> Out1/1
  Demux1/7 -> Mux/7  "omega_VSP2"
  Demux1/6 -> Mux/6  "omega_VSP1"
  Demux1/5 -> Mux/5  "alpha_VSP2"
  Demux1/4 -> Mux/4  "alpha_VSP1"
  Demux1/3 -> Mux/3  "u_VSP2"
  Demux1/2 -> Mux/2  "u_VSP1"
  Demux1/1 -> Mux/1  "u_BT"
  In1/1 -> Demux1/1

== system Sim_13_forh/Controller/SIXAIS/Sixais Controller Not Simulated in Simulink ==
  In1 : Inport
  In2 : Inport  Port=2
  In3 : Inport  Port=3
  In4 : Inport  Port=4
  In5 : Inport  Port=5
  In6 : Inport  Port=6
  In7 : Inport  Port=7
  Mux1 : Mux  Inputs=7
  Out1 : Outport  VectorParamsAs1DForOutWhenUnconnected=off
  wires:
  In4/1 -> Mux1/4
  In5/1 -> Mux1/5
  In6/1 -> Mux1/6
  In3/1 -> Mux1/3
  In1/1 -> Mux1/1
  In2/1 -> Mux1/2
  Mux1/1 -> Out1/1
  In7/1 -> Mux1/7

== system Sim_13_forh/Controller/Subsystem/1//|p_d'| ==
  s : Inport
  switch : Inport  Port=2
  Elipse : MATLAB Function  TreatAsAtomicUnit=on
  Straight line : MATLAB Function  TreatAsAtomicUnit=on
  Switch : Switch  Criteria=u2 > Threshold
  1/|p_d'| : Outport
  wires:
  s/1 -> Elipse/1(s)
  Elipse/1(y) -> Switch/3
  Switch/1 -> 1/|p_d'|/1
  Straight line/1(y) -> Switch/1
  switch/1 -> Switch/2

== system Sim_13_forh/Controller/Subsystem/Final_Tau_Computation ==
  alpha_1 : Inport
  alpha_1_dot : Inport  Port=2
  nu_hat : Inport  Port=3
  Gain : Gain  Gain=K_v  Multiplication=Matrix(K*u)
  Gain1 : Gain  Gain=M  Multiplication=Matrix(K*u)
  Gain2 : Gain  Gain=D  Multiplication=Matrix(K*u)
  Sum : Sum  Inputs=-+|
  Sum1 : Sum  Inputs=++-
  Tau : Outport
  wires:
  nu_hat/1 -> Sum/2
  alpha_1/1 -> Gain2/1, Sum/1
  Sum/1 -> Gain/1  "z_2"
  Sum1/1 -> Tau/1
  Gain/1 -> Sum1/3
  alpha_1_dot/1 -> Gain1/1
  Gain1/1 -> Sum1/1
  Gain2/1 -> Sum1/2

== system Sim_13_forh/Controller/Subsystem/U_s(s) ==
  s : Inport
  switch : Inport  Port=2
  Eliptical : MATLAB Function  TreatAsAtomicUnit=on
  Straight line : MATLAB Function  TreatAsAtomicUnit=on
  Switch : Switch  Criteria=u2 > Threshold
  U_s : Outport
  wires:
  Straight line/1(y) -> Switch/1
  Switch/1 -> U_s/1
  Eliptical/1(y) -> Switch/3
  s/1 -> Eliptical/1(s)
  switch/1 -> Switch/2

== system Sim_13_forh/Controller/Subsystem/U_s(s)' ==
  s : Inport
  "switch " : Inport  Port=2
  Constant : Constant  Value=0
  MATLAB Function : MATLAB Function  TreatAsAtomicUnit=on
  Switch : Switch  Criteria=u2 > Threshold
  U_s' : Outport
  wires:
  s/1 -> MATLAB Function/1(s)
  MATLAB Function/1(U_sf) -> Switch/3
  Switch/1 -> U_s'/1
  Constant/1 -> Switch/1
  "switch "/1 -> Switch/2

== system Sim_13_forh/Controller/Subsystem/alpha_1, z_1 - explicit  ==
  eta : Inport
  eta_d(s) : Inport  Port=2
  eta_d(s)' : Inport  Port=3
  U_s : Inport  Port=4
  Gain : Gain  Gain=-K_p
  Product : Product
  Product1 : Product  Inputs=3
  Rotation Matrix : MATLAB Function  TreatAsAtomicUnit=on
  Selector : Selector  InputPortWidth=3  IndexOptions=Index vector (dialog)  Indices=[3]  OutputSizes=1
  Sum : Sum  Inputs=|+-
  Sum1 : Sum  Inputs=|++
  Transpose : Math  Operator=transpose  SignedPower=off  SaturateOnIntegerOverflow=on
  alpha_1 : Outport
  z_1 : Outport  Port=2
  wires:
  eta/1 -> Sum/1, Selector/1
  Selector/1 -> Rotation Matrix/1(psi)
  eta_d(s)/1 -> Sum/2
  Sum/1 -> Product/2
  Rotation Matrix/1(R_psi) -> Transpose/1
  Product/1 -> Gain/1, z_1/1
  Gain/1 -> Sum1/1
  Sum1/1 -> alpha_1/1
  Transpose/1 -> Product1/1, Product/1
  Product1/1 -> Sum1/2
  eta_d(s)'/1 -> Product1/2
  U_s/1 -> Product1/3

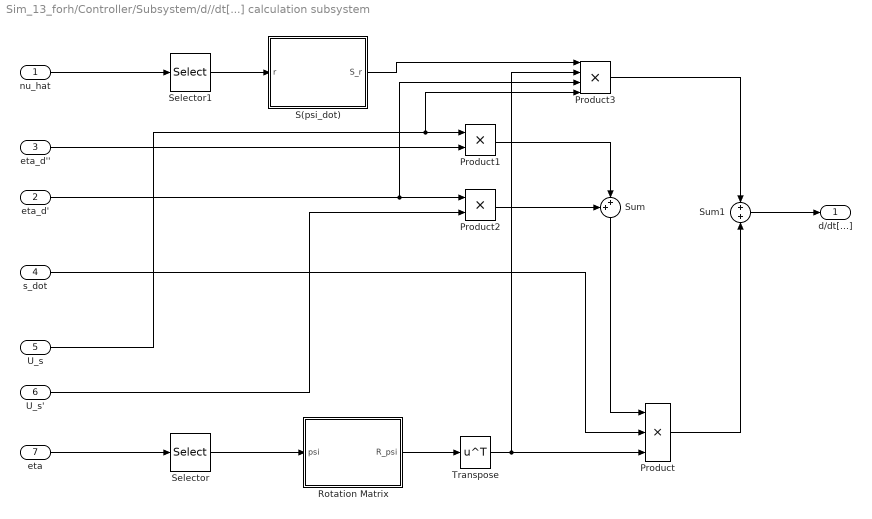
== system Sim_13_forh/Controller/Subsystem/d//dt[...] calculation subsystem ==
  nu_hat : Inport
  eta_d' : Inport  Port=2
  eta_d'' : Inport  Port=3
  s_dot : Inport  Port=4
  U_s : Inport  Port=5
  "U_s' " : Inport  Port=6
  "eta " : Inport  Port=7
  Product : Product  Inputs=3
  Product1 : Product
  Product2 : Product
  Product3 : Product  Inputs=4
  Rotation Matrix : MATLAB Function  TreatAsAtomicUnit=on
  S(psi_dot) : MATLAB Function  TreatAsAtomicUnit=on
  Selector : Selector  InputPortWidth=3  IndexOptions=Index vector (dialog)  Indices=[3]  OutputSizes=1
  Selector1 : Selector  InputPortWidth=3  IndexOptions=Index vector (dialog)  Indices=[3]  OutputSizes=1
  Sum : Sum  Inputs=++|
  Sum1 : Sum
  Transpose : Math  Operator=transpose  SignedPower=off  SaturateOnIntegerOverflow=on
  d/dt[...] : Outport
  wires:
  "eta "/1 -> Selector/1
  Selector/1 -> Rotation Matrix/1(psi)
  Rotation Matrix/1(R_psi) -> Transpose/1
  Transpose/1 -> Product3/2, Product/3
  s_dot/1 -> Product/2
  eta_d''/1 -> Product1/2
  U_s/1 -> Product3/4, Product1/1
  Sum/1 -> Product/1
  Product1/1 -> Sum/2
  eta_d'/1 -> Product3/3, Product2/1
  "U_s' "/1 -> Product2/2
  Product2/1 -> Sum/1
  nu_hat/1 -> Selector1/1
  Selector1/1 -> S(psi_dot)/1("r ")
  S(psi_dot)/1(S_r) -> Product3/1
  Product/1 -> Sum1/2
  Product3/1 -> Sum1/1
  Sum1/1 -> d/dt[...]/1

== system Sim_13_forh/Controller/Subsystem/eta_d''(s) ==
  s : Inport
  switch : Inport  Port=2
  Constant : Constant  Value=[0 0 0]'
  MATLAB Function : MATLAB Function  TreatAsAtomicUnit=on
  Switch : Switch  Criteria=u2 > Threshold
  "eta_d''(s) " : Outport
  wires:
  s/1 -> MATLAB Function/1(s)
  MATLAB Function/1(y) -> Switch/3
  Switch/1 -> "eta_d''(s) "/1
  Constant/1 -> Switch/1
  switch/1 -> Switch/2

== system Sim_13_forh/Controller/Subsystem/eta_d'(s) ==
  s : Inport
  switch : Inport  Port=2
  MATLAB Function : MATLAB Function  TreatAsAtomicUnit=on
  MATLAB Function1 : MATLAB Function  TreatAsAtomicUnit=on
  Switch : Switch  Criteria=u2 > Threshold
  Out1 : Outport
  wires:
  s/1 -> MATLAB Function/1(s)
  MATLAB Function/1(y) -> Switch/3
  Switch/1 -> Out1/1
  MATLAB Function1/1(y) -> Switch/1
  switch/1 -> Switch/2

== system Sim_13_forh/Controller/Subsystem/eta_d(s) ==
  s : Inport
  switch : Inport  Port=2
  Eliptical path : MATLAB Function  TreatAsAtomicUnit=on
  Straight line : MATLAB Function  TreatAsAtomicUnit=on
  Switch : Switch  Criteria=u2 > Threshold
  "eta_d''(s) " : Outport
  wires:
  s/1 -> Straight line/1(s), Eliptical path/1(s)
  Eliptical path/1(y) -> Switch/3
  Switch/1 -> "eta_d''(s) "/1
  Straight line/1(y) -> Switch/1
  switch/1 -> Switch/2

== system Sim_13_forh/Controller/Subsystem/z_1_dot subsystem  ==
  eta_d : Inport
  eta_d' : Inport  Port=2
  eta : Inport  Port=3
  s_dot : Inport  Port=4
  nu_hat : Inport  Port=5
  Product : Product  Inputs=3
  Product1 : Product  Inputs=3
  Rotation Matrix : MATLAB Function  TreatAsAtomicUnit=on
  S(psi_dot) : MATLAB Function  TreatAsAtomicUnit=on
  Selector : Selector  InputPortWidth=3  IndexOptions=Index vector (dialog)  Indices=[3]  OutputSizes=1
  Selector1 : Selector  InputPortWidth=3  IndexOptions=Index vector (dialog)  Indices=[3]  OutputSizes=1
  Sum : Sum  Inputs=-+|
  Sum1 : Sum  Inputs=+++
  Transpose : Math  Operator=transpose  SignedPower=off  SaturateOnIntegerOverflow=on
  Transpose1 : Math  Operator=transpose  SignedPower=off  SaturateOnIntegerOverflow=on
  z_1_dot : Outport
  wires:
  nu_hat/1 -> Sum1/3, Selector/1
  Selector/1 -> S(psi_dot)/1("r ")
  eta/1 -> Selector1/1, Sum/2
  eta_d/1 -> Sum/1
  Selector1/1 -> Rotation Matrix/1(psi)
  Rotation Matrix/1(R_psi) -> Transpose1/1
  Sum/1 -> Product/1
  S(psi_dot)/1(S_r) -> Transpose/1
  Transpose/1 -> Product/3
  Sum1/1 -> z_1_dot/1
  Product/1 -> Sum1/2
  s_dot/1 -> Product1/2
  eta_d'/1 -> Product1/1
  Product1/1 -> Sum1/1
  Transpose1/1 -> Product/2, Product1/3

== system Sim_13_forh/Nonlinear Observer and Dead Reckoning/Dead Reckoning/Pose ==
  eta : Inport
  Demux : Demux  Outputs=3
  Gain : Gain  Gain=1/1000
  Gain1 : Gain  Gain=1/1000
  Gain2 : Gain  Gain=180/pi
  Gain3 : Gain  Gain=pi/180
  MATLAB Function : MATLAB Function  TreatAsAtomicUnit=on
  Memory : Memory
  Mux : Mux  Inputs=3
  Wrap2psi : MATLAB Function  TreatAsAtomicUnit=on
  QTM : Outport  VectorParamsAs1DForOutWhenUnconnected=off
  wires:
  Demux/2 -> Gain1/1  "y_m"
  Demux/3 -> Gain3/1  "psi_m"
  Demux/1 -> Gain/1  "x_m"
  Mux/1 -> QTM/1
  eta/1 -> Demux/1
  ? -> Wrap2psi/1(u)
  Wrap2psi/1(yQualisus) -> Gain2/1
  Gain/1 -> Mux/1
  Gain1/1 -> Mux/2
  Gain3/1 -> MATLAB Function/1(psi)
  MATLAB Function/1(psi_out) -> Memory/1, Mux/3
  Memory/1 -> MATLAB Function/2(psi_old)

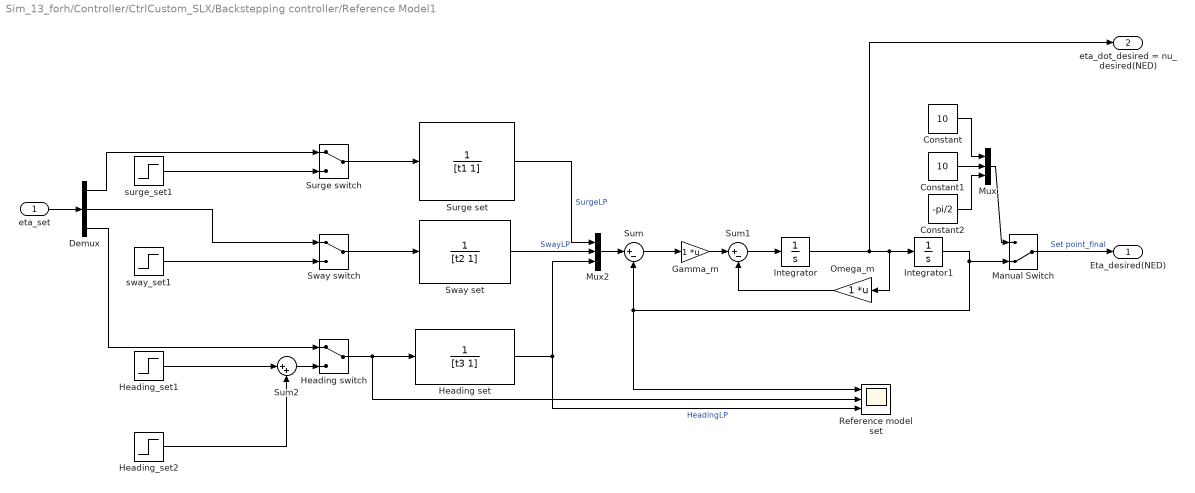
== system Sim_13_forh/Controller/CtrlCustom_SLX/Backstepping controller/Reference Model1 ==
  "eta_set " : Inport
  Constant : Constant  Value=10
  Constant1 : Constant  Value=10
  Constant2 : Constant  Value=-pi/2
  Demux : Demux  Outputs=3
  "Gamma_m " : Gain  Multiplication=Matrix(K*u)
  Heading set : TransferFcn  Denominator=[t3 1]
  "Heading switch " : ManualSwitch
  Heading_set1 : Step  Time=100  After=-pi/4  SampleTime=0
  Heading_set2 : Step  Time=800  After=pi/4  SampleTime=0
  Integrator : Integrator
  Integrator1 : Integrator
  Manual Switch : ManualSwitch  CurrentSetting=0
  Mux : Mux  Inputs=3
  Mux2 : Mux  Inputs=3
  Omega_m : Gain  Multiplication=Matrix(K*u)
  "Reference model set " : Scope  NumInputPorts=3
  Sum : Sum  Inputs=|+-
  Sum1 : Sum  Inputs=|+-
  Sum2 : Sum  Inputs=|++
  Surge set : TransferFcn  Denominator=[t1 1]
  "Surge switch " : ManualSwitch
  Sway set : TransferFcn  Denominator=[t2 1]
  Sway switch : ManualSwitch
  "surge_set1 " : Step  Time=0  After=50  SampleTime=0
  sway_set1 : Step  Time=100  After=0  SampleTime=0
  Eta_desired(NED) : Outport  VectorParamsAs1DForOutWhenUnconnected=off
  eta_dot_desired = nu_desired(NED) : Outport  Port=2  VectorParamsAs1DForOutWhenUnconnected=off
  wires:
  Sum1/1 -> Integrator/1
  Surge set/1 -> Mux2/1  "SurgeLP"
  Sway set/1 -> Mux2/2  "SwayLP"
  Sum/1 -> "Gamma_m "/1
  Mux2/1 -> Sum/1
  Omega_m/1 -> Sum1/2
  Heading set/1 -> Mux2/3, "Reference model set "/3  "HeadingLP"
  "Gamma_m "/1 -> Sum1/1
  "Heading switch "/1 -> Heading set/1, "Reference model set "/2
  Integrator1/1 -> Manual Switch/2, "Reference model set "/1, Sum/2
  "eta_set "/1 -> Demux/1
  Demux/1 -> "Surge switch "/1
  "surge_set1 "/1 -> "Surge switch "/2
  "Surge switch "/1 -> Surge set/1
  Sway switch/1 -> Sway set/1
  sway_set1/1 -> Sway switch/2
  Demux/2 -> Sway switch/1
  Demux/3 -> "Heading switch "/1
  Heading_set1/1 -> Sum2/1
  Mux/1 -> Manual Switch/1
  Manual Switch/1 -> Eta_desired(NED)/1  "Set point_final"
  Constant/1 -> Mux/1
  Constant1/1 -> Mux/2
  Constant2/1 -> Mux/3
  Integrator/1 -> eta_dot_desired = nu_desired(NED)/1, Omega_m/1, Integrator1/1
  Sum2/1 -> "Heading switch "/2
  Heading_set2/1 -> Sum2/2

== system Sim_13_forh/Controller/CtrlCustom_SLX/Backstepping controller/alpha_1, z_1 - explicit  ==
  eta : Inport
  eta_d(s) : Inport  Port=2
  eta_d(s)' : Inport  Port=3
  U_s : Inport  Port=4
  Gain : Gain  Gain=-K_p
  Product : Product
  Product1 : Product  Inputs=3
  Rotation Matrix : MATLAB Function  TreatAsAtomicUnit=on
  Selector : Selector  InputPortWidth=3  IndexOptions=Index vector (dialog)  Indices=[3]  OutputSizes=1
  Sum : Sum  Inputs=|+-
  Sum1 : Sum  Inputs=|++
  Transpose : Math  Operator=transpose  SignedPower=off  SaturateOnIntegerOverflow=on
  alpha_1 : Outport
  z_1 : Outport  Port=2
  wires:
  eta/1 -> Sum/1, Selector/1
  Selector/1 -> Rotation Matrix/1(psi)
  eta_d(s)/1 -> Sum/2
  Sum/1 -> Product/2
  Rotation Matrix/1(R_psi) -> Transpose/1
  Product/1 -> Gain/1, z_1/1
  Gain/1 -> Sum1/1
  Sum1/1 -> alpha_1/1
  Transpose/1 -> Product1/1, Product/1
  Product1/1 -> Sum1/2
  eta_d(s)'/1 -> Product1/2
  U_s/1 -> Product1/3

== system Sim_13_forh/Controller/DP_Ctrl/Backstepping controller/1//|p_d'| ==
  s : Inport
  switch : Inport  Port=2
  Elipse : MATLAB Function  TreatAsAtomicUnit=on
  Straight line : MATLAB Function  TreatAsAtomicUnit=on
  Switch : Switch  Criteria=u2 > Threshold
  1/|p_d'| : Outport
  wires:
  s/1 -> Elipse/1(s)
  Elipse/1(y) -> Switch/3
  Switch/1 -> 1/|p_d'|/1
  Straight line/1(y) -> Switch/1
  switch/1 -> Switch/2
